simulink model "v00_0A_0E"  (R2022b)
settings: Solver=FixedStepDiscrete  StartTime=0.0  StopTime=8000  FixedStep=SampleTime  MaxStep=Contactors_StepTime_msec  RelTol=1e-3  EnableMultiTasking=on
undefined symbols (not defined in the file): A_to_mA, BalancingTempGroup, canChannel, CapacityFactor, CC_Inputs, CellSOC, ChargeState, ContactorsFlags, DiscIntNeverNeededParam, gEN_Contactors_StepTime_msec, Ion, isDynamicCurrentEn, Lithium, maxAllowedImbalance, nCells_parallel, nCells_series, nCellTempGrps, PermanentFailRecoveryTrigger, ProtectionFlags, RBal_ohm, SampleTime, sigbuilder_block, StLineEq_varA, StLineEq_varB, TempSelectForDCL, Thresholds, V_to_mV
libraries: simulink x32, spsIdealSwitchLib x21, spsBatteryLib x20, spsSeriesRLCBranchLib x20, spsVoltageMeasurementLib x20, canmsglib x4, canlib x3, dspstat3 x2, spspowerguiLib x2, spsControlledCurrentSourceLib x1, spsCurrentMeasurementLib x1
(part 6 of 7)

== stateflow chart v00_0A_0E/Protection/CurrentVoltageTemperature_Statemachine ==
  state ThermalRunaway [parallel]
    settings: executionOrder=6
    state ThermalRunaway_Warning
      entry:
      ThermalRunaway = ProtectionFlags.Warning;
    state ThermalRunaway_NoError
      entry:
      ThermalRunaway = ProtectionFlags.NoError;
    state ThermalRunaway_PermanentFail
      entry:
      ThermalRunaway = ProtectionFlags.PermanentFail;
    state ThermalRunaway_Error
      entry:
      ThermalRunaway = ProtectionFlags.Error;
    ThermalRunaway_NoError -> ThermalRunaway_Warning : [duration((TempChange_C>=Thresholds.Protections_MaxAllowedTempChange_C && DataPipeline.TemperatureSenseBus(1).T_max >Thresholds.Protections_MaxOperatingTemp_C),msec) >=Thresholds.ThermalRunawayWarningTimeout_msec]
    (default) -> ThermalRunaway_NoError
    ThermalRunaway_Warning -> ThermalRunaway_Error : [duration((TempChange_C >= Thresholds.Protections_MaxAllowedTempChange_C && DataPipeline.TemperatureSenseBus(1).T_max > Thresholds.Protections_MaxOperatingTemp_C),msec) >=Thresholds.ThermalRunawayErrorTimeout_msec]
    ThermalRunaway_Error -> ThermalRunaway_PermanentFail : [duration((ThermalRunaway == ProtectionFlags.Error),msec) >=Thresholds.ThermalRunawayErrorTimeout_msec]
  state SuddenVoltageDrop [parallel]
    settings: executionOrder=10
    state Lobby
      entry:
      SuddenVoltageDrop = ProtectionFlags.NoError;
    state Error
      entry:
      SuddenVoltageDrop = ProtectionFlags.Error;
    (default) -> SuddenVoltageDrop.Lobby
    SuddenVoltageDrop.Lobby -> SuddenVoltageDrop.Error : [duration((VoltageDrop_mV >= Thresholds.Protections_SuddenVoltageDrop_mV_by_time),msec) >= Thresholds.SuddenVoltageDropTimeout_msec]
    SuddenVoltageDrop.Error -> SuddenVoltageDrop.Lobby : [duration((VoltageDrop_mV < Thresholds.Protections_SuddenVoltageDrop_mV_by_time),msec) >= Thresholds.SuddenVoltageDropTimeout_msec]
  state Current_Protection [parallel]
    settings: executionOrder=3
    state OCD_Error
      entry:
      OCDFlag = ProtectionFlags.Error;
      OCCFlag = ProtectionFlags.NoError;
    state Lobby
      entry:
      OCD_Warning_mA = Thresholds.Protections_OCD_Warning_mA;
      OCD_Error_mA = Thresholds.Protections_OCD_Error_mA;
      OCC_Warning_mA = Thresholds.Protections_OCC_Warning_mA;
      OCC_Error_mA = Thresholds.Protections_OCC_Error_mA;
    state OverCurrent_DynamicCurrentLimits
      entry:
      eFuseChargeFlag= ProtectionFlags.NoError;
      eFuseDischargeFlag= ProtectionFlags.NoError;
      during:
      i2tCalculation_DCL;
      DCL_Current_A = (single(DataPipeline.isChargeEn) * single(DataPipeline.DCL_ChargingCurrent_A))+(single(~DataPipeline.isChargeEn) * single(DataPipeline.DCL_DisChargingCurrent_A));
      state i2tCalculation_DCL [function]
        (default) -> (junction 1122) : % IfStatement
        (junction 1122) -> (junction 1125) [order 1] : [i2t_Calculated_A2sec >0]
        (junction 1125) -> (junction 1123) : {CurrentDiff_A = single(abs(DataPipeline.Current_mA)/1000) - single(abs(DCL_Current_A));
            | i2t_Calculated_A2sec = i2t_Calculated_A2sec - (CurrentDiff_A * CurrentDiff_A * DataPipeline.LoopTimer_SOC_msec/1000);}
        (junction 1122) -> (junction 1124) [order 2] : {i2t_Calculated_A2sec = single(0);}
        (junction 1123) -> (junction 1124)
        (junction 1124) -> (junction 1126)
    state OCD_Warning
      entry:
      OCDFlag = ProtectionFlags.Warning;
      OCCFlag = ProtectionFlags.NoError;
    state OCD_Recovery
      entry:
      OCDFlag = ProtectionFlags.Recovery;
      OCCFlag = ProtectionFlags.NoError;
    state No_Error_Current
      entry:
      OCDFlag = ProtectionFlags.NoError;
      OCCFlag = ProtectionFlags.NoError;
    state eFuse_Melting
      du:  eFuseWarning;
      DCL_Current_A = single((single(DataPipeline.isChargeEn) * single(DataPipeline.DCL_ChargingCurrent_A))+(single(~DataPipeline.isChargeEn) * single(DataPipeline.DCL_DisChargingCurrent_A)));
      CurrentDiff_A = single(abs(DataPipeline.Current_mA)/1000) - single(abs(DCL_Current_A));
      i2t_Calculated_A2sec = i2t_Calculated_A2sec + (CurrentDiff_A * CurrentDiff_A * DataPipeline.LoopTimer_SOC_msec/1000);
      % i2t_Calculated_A2sec = 110000;
      state eFuseWarning [function]
        (default) -> (junction 1136) : % eFuseDuringCharge&Discharge
        (junction 1136) -> (junction 1135) [order 1] : [DataPipeline.VCU.isChargerConnected == 1]
        (junction 1136) -> (junction 1139) [order 2] : {eFuseDischargeFlag= ProtectionFlags.Warning;}
        (junction 1135) -> (junction 1132) : {eFuseChargeFlag= ProtectionFlags.Warning;}
        (junction 1132) -> (junction 1139)
        (junction 1139) -> (junction 1138)
    state OCC_Warning
      entry:
      OCCFlag = ProtectionFlags.Warning;
      OCDFlag = ProtectionFlags.NoError;
    state OCC_Recovery
      entry:
      OCCFlag = ProtectionFlags.Recovery;
      OCDFlag = ProtectionFlags.NoError;
    state OCC_Error
      entry:
      OCCFlag = ProtectionFlags.Error;
      OCDFlag = ProtectionFlags.NoError;
    state eFuse_Melted
      entry:
      i2t_Calculated_A2sec = single(0);
      eFuseError;
      state eFuseError [function]
        (default) -> (junction 1146) : % eFuseDuringCharge&Discharge
        (junction 1146) -> (junction 1147) [order 1] : [DataPipeline.VCU.isChargerConnected == 1]
        (junction 1146) -> (junction 1148) [order 2] : {eFuseDischargeFlag= ProtectionFlags.Error;}
        (junction 1147) -> (junction 1149) : {eFuseChargeFlag= ProtectionFlags.Error;}
        (junction 1149) -> (junction 1148)
        (junction 1148) -> (junction 1153)
    state PermanentFail_eFuse
      entry:
      eFusePermanentFail;
      state eFusePermanentFail [function]
        (default) -> (junction 1167) : % eFuseDuringCharge&Discharge
        (junction 1167) -> (junction 1161) [order 1] : [DataPipeline.VCU.isChargerConnected == 1]
        (junction 1167) -> (junction 1170) [order 2] : {eFuseDischargeFlag= ProtectionFlags.PermanentFail;}
        (junction 1161) -> (junction 1164) : {eFuseChargeFlag= ProtectionFlags.PermanentFail;}
        (junction 1164) -> (junction 1170)
        (junction 1170) -> (junction 1165)
    (default) -> Current_Protection.Lobby
    OCD_Recovery -> OCD_Error [order 2] : [(duration(abs(DataPipeline.Current_mA) >= OCD_Error_mA, msec) > Thresholds.Protections_OCD_WarningTimeout_msec)]
    OCD_Warning -> OCD_Error [order 1] : [(duration(abs(DataPipeline.Current_mA) >= OCD_Error_mA, msec) > Thresholds.Protections_OCD_WarningTimeout_msec)]
    OCD_Error -> OCD_Recovery : [after(Thresholds.Protections_OCD_ErrorTimeout_msec, msec)]
    Current_Protection.Lobby -> No_Error_Current [order 2] : [DataPipeline.isDynamicCurrentEn == 0 ]
    Current_Protection.Lobby -> OverCurrent_DynamicCurrentLimits [order 1] : [DataPipeline.isDynamicCurrentEn == 1 ]
    No_Error_Current -> OCD_Warning [order 1] : [DataPipeline.VCU.isChargerConnected == 0 && duration(abs(DataPipeline.Current_mA) >= OCD_Warning_mA, msec) > Thresholds.Protections_OCD_NoErrorTimeout_msec]
    OCD_Warning -> No_Error_Current [order 2] : [duration(abs(DataPipeline.Current_mA) <= OCD_Warning_mA, msec) > Thresholds.Protections_OCD_WarningTimeout_msec]
    OCD_Recovery -> No_Error_Current [order 1] : [duration(abs(DataPipeline.Current_mA) <= OCD_Error_mA, msec) > Thresholds.Protections_OCD_RecoveryTimeout_msec]
    eFuse_Melted -> OverCurrent_DynamicCurrentLimits [order 1] : [after(Thresholds.i2tTimeout_msec,msec)]
    OCC_Recovery -> No_Error_Current [order 1] : [duration(abs(DataPipeline.Current_mA) <= OCC_Error_mA, msec) > Thresholds.Protections_OCC_RecoveryTimeout_msec]
    No_Error_Current -> OCC_Warning [order 2] : [DataPipeline.VCU.isChargerConnected == 1 && duration(abs(DataPipeline.Current_mA) >= OCC_Warning_mA,msec) > Thresholds.Protections_OCC_NoErrorTimeout_msec]
    OCC_Warning -> No_Error_Current [order 2] : [duration(abs(DataPipeline.Current_mA) <= OCC_Warning_mA, msec) > Thresholds.Protections_OCC_WarningTimeout_msec]
    OverCurrent_DynamicCurrentLimits -> eFuse_Melting : [duration((abs(DataPipeline.Current_mA)/1000) > abs(DCL_Current_A),msec) >= Thresholds.i2tTimeout_msec]
    eFuse_Melting -> OverCurrent_DynamicCurrentLimits [order 1] : [duration((abs(DataPipeline.Current_mA)/1000) < abs(DCL_Current_A),msec) >= Thresholds.i2tTimeout_msec]
    OCC_Warning -> OCC_Error [order 1] : [duration(abs(DataPipeline.Current_mA) >= OCC_Error_mA, msec) > Thresholds.Protections_OCC_WarningTimeout_msec]
    OCC_Error -> OCC_Recovery : [after(Thresholds.Protections_OCC_ErrorTimeout_msec, msec)]
    OCC_Recovery -> OCC_Error [order 2] : [duration(abs(DataPipeline.Current_mA) >= OCC_Error_mA, msec) > Thresholds.Protections_OCC_WarningTimeout_msec]
    eFuse_Melting -> eFuse_Melted [order 2] : [duration(((i2t_Calculated_A2sec >= DataPipeline.i2t_ChargingCurrent_A2sec && DataPipeline.VCU.isChargerConnected == 1)), msec)>= Thresholds.eFuseMeltingTimeout_msec || duration(((i2t_Calculated_A2sec >= DataPipeline.i2t_DisChargingCurrent_A2sec && DataPipeline.VCU.isChargerConnected == 0)), msec)>= Thresholds.eFuseMeltingTimeout_msec]
        | {eFuseMeltCount = eFuseMeltCount + 1;}
    eFuse_Melted -> PermanentFail_eFuse [order 2] : [eFuseMeltCount >= Thresholds.PermanentFailCounts_eFuse]
  state Voltage_Protection [parallel]
    settings: executionOrder=2
    state UV_Error
      entry:
      UVFlag = ProtectionFlags.Error;
      OVFlag = ProtectionFlags.NoError;
    state UV_Recovery
      entry:
      UVFlag = ProtectionFlags.Recovery;
      OVFlag = ProtectionFlags.NoError;
    state UV_Warning
      entry:
      UVFlag = ProtectionFlags.Warning;
      OVFlag = ProtectionFlags.NoError;
    state No_Error_Voltage
      entry:
      UVFlag = ProtectionFlags.NoError;
      OVFlag = ProtectionFlags.NoError;
    state OV_Recovery
      entry:
      OVFlag = ProtectionFlags.Recovery;
      UVFlag = ProtectionFlags.NoError;
    state OV_Warning
      entry:
      OVFlag = ProtectionFlags.Warning;
      UVFlag = ProtectionFlags.NoError;
    state OV_Error
      entry:
      OVFlag = ProtectionFlags.Error;
      UVFlag = ProtectionFlags.NoError;
    UV_Recovery -> UV_Error [order 2] : [duration((DataPipeline.VoltageSenseBus.mV_min < Thresholds.Protections_UV_Error_mV), msec) > Thresholds.Protections_UV_WarningTimeout_msec]
    UV_Warning -> UV_Error [order 2] : [duration((DataPipeline.VoltageSenseBus.mV_min < Thresholds.Protections_UV_Error_mV && DataPipeline.VCU.isChargerConnected == 0), msec) > Thresholds.Protections_UV_WarningTimeout_msec]
    UV_Error -> UV_Recovery : [(duration((DataPipeline.VoltageSenseBus.mV_min > Thresholds.Protections_UV_Error_mV  || DataPipeline.VCU.isChargerConnected ==1), msec) > Thresholds.Protections_UV_ErrorTimeout_msec)]
    No_Error_Voltage -> UV_Warning [order 1] : [(duration(DataPipeline.VoltageSenseBus.mV_min <= Thresholds.Protections_UV_Warning_mV, msec) > Thresholds.Protections_UV_NoErrorTimeout_msec)]
    UV_Warning -> No_Error_Voltage [order 1] : [(duration((DataPipeline.VoltageSenseBus.mV_min > Thresholds.Protections_UV_Warning_mV), msec) > Thresholds.Protections_OV_WarningTimeout_msec)]
    UV_Recovery -> No_Error_Voltage [order 1] : [duration((DataPipeline.VoltageSenseBus.mV_min >= Thresholds.Protections_UV_Recovery_mV || DataPipeline.VCU.isChargerConnected ==1),msec) > Thresholds.Protections_UV_RecoveryTimeout_msec]
    (default) -> No_Error_Voltage
    No_Error_Voltage -> OV_Warning [order 2] : [duration(DataPipeline.VoltageSenseBus.mV_max >= Protections_OV_Warning_mV && (DataPipeline.VCU.isChargerConnected==1 || DataPipeline.Current_mA>0), msec) > Thresholds.Protections_OV_NoErrorTimeout_msec]
    OV_Recovery -> No_Error_Voltage [order 1] : [duration((DataPipeline.VoltageSenseBus.mV_max <= Protections_OV_Recovery_mV || DataPipeline.VCU.isChargerConnected ==0), msec) > Thresholds.Protections_OV_RecoveryTimeout_msec]
    OV_Warning -> No_Error_Voltage [order 1] : [(duration((DataPipeline.VoltageSenseBus.mV_max < Protections_OV_Warning_mV), msec) > Thresholds.Protections_OV_WarningTimeout_msec)]
    OV_Error -> OV_Recovery : [(duration((DataPipeline.VoltageSenseBus.mV_max < Protections_OV_Error_mV || DataPipeline.VCU.isChargerConnected ==0), msec) > Thresholds.Protections_OV_ErrorTimeout_msec)]
    OV_Recovery -> OV_Error [order 2] : [(duration((DataPipeline.VoltageSenseBus.mV_max > Protections_OV_Error_mV), msec) > Thresholds.Protections_OV_WarningTimeout_msec)]
    OV_Warning -> OV_Error [order 2] : [duration(DataPipeline.VoltageSenseBus.mV_max > Protections_OV_Error_mV && (DataPipeline.VCU.isChargerConnected ==1 || DataPipeline.Current_mA>0), msec) > Thresholds.Protections_OV_WarningTimeout_msec]
  state TemperatureGradient [parallel]
    settings: executionOrder=7
    state Lobby
      entry:
      TemperatureGradient = ProtectionFlags.NoError;
    state Error
      entry:
      TemperatureGradient = ProtectionFlags.Error;
    (default) -> TemperatureGradient.Lobby
    TemperatureGradient.Error -> TemperatureGradient.Lobby : [duration(DataPipeline.DeltaTemperatureGroup1_C < Thresholds.Protections_MaxAllowedTempGradientGroup1_C, msec) >= Thresholds.TemperatureGradientTimeout_msec]
    TemperatureGradient.Lobby -> TemperatureGradient.Error : [duration(DataPipeline.DeltaTemperatureGroup1_C >= Thresholds.Protections_MaxAllowedTempGradientGroup1_C, msec) >= Thresholds.TemperatureGradientTimeout_msec]
  state OverallState [parallel]
    settings: executionOrder=12
    state Lobby
      entry: TempOverallState = ProtectionFlags.NoError;
    state Warning
      entry: TempOverallState = ProtectionFlags.Warning;
    state Error
      entry: TempOverallState = ProtectionFlags.Error;
    state Recovery
      entry:  TempOverallState = ProtectionFlags.Recovery;
    (default) -> OverallState.Lobby
    Warning -> OverallState.Lobby [order 2] : [FlagGroup1 == 0 && FlagGroup2 == 0]
    OverallState.Lobby -> Warning : [FlagGroup1 >= 1 || FlagGroup2 >= 1]
    OverallState.Error -> OverallState.Lobby [order 2] : [FlagGroup1 == 0 && FlagGroup2 == 0]
    Recovery -> OverallState.Lobby : [FlagGroup1 == 0 && FlagGroup2 == 0]
    Warning -> OverallState.Error [order 1] : [FlagGroup1 >= 2 || FlagGroup2 >= 2]
    OverallState.Error -> Recovery [order 1] : [(FlagGroup1 == 3 && FlagGroup2 == 0)||(FlagGroup1 == 0 && FlagGroup2==3)]
  state HighImbalanceFlag [parallel]
    settings: executionOrder=8
    state Lobby
      entry:
      HighImbalanceFlag = ProtectionFlags.NoError;
    state Error
      entry:
      HighImbalanceFlag = ProtectionFlags.Error;
    (default) -> HighImbalanceFlag.Lobby
    HighImbalanceFlag.Lobby -> HighImbalanceFlag.Error : [duration((DataPipeline.VoltageSenseBus.VoltageDelta_mV >= Thresholds.Protections_HighImbalanceError_mV),msec) >= Thresholds.HighImbalanceFlagTimeout_msec]
    HighImbalanceFlag.Error -> HighImbalanceFlag.Lobby : [duration((DataPipeline.VoltageSenseBus.VoltageDelta_mV < Thresholds.Protections_HighImbalanceError_mV),msec) >= Thresholds.HighImbalanceFlagTimeout_msec]
  state ErrorDetect [parallel]
    settings: executionOrder=11
    state Lobby
      entry:
      ErrorDetect = ProtectionFlags.NoError;
    state Error
      entry:
      ErrorDetect = ProtectionFlags.Error;
    (default) -> ErrorDetect.Lobby
    ErrorDetect.Lobby -> ErrorDetect.Error : [ThermalRunaway==ProtectionFlags.Error||TemperatureGradient==ProtectionFlags.Error||HighImbalanceFlag==ProtectionFlags.Error||ShortCircuitDetect==ProtectionFlags.Error||SuddenVoltageDrop == ProtectionFlags.Error||TempOverallState==ProtectionFlags.Error||OCCFlag==ProtectionFlags.Error||OCDFlag==ProtectionFlags.Error||UVFlag==ProtectionFlags.Error||OVFlag==ProtectionFlags.Error ||eFuseChargeFlag==ProtectionFlags.Error || eFuseDischargeFlag==ProtectionFlags.Error]
    ErrorDetect.Error -> ErrorDetect.Lobby : [ThermalRunaway~=ProtectionFlags.Error && TemperatureGradient~=ProtectionFlags.Error && HighImbalanceFlag~=ProtectionFlags.Error && ShortCircuitDetect~=ProtectionFlags.Error && SuddenVoltageDrop~=ProtectionFlags.Error && TempOverallState~=ProtectionFlags.Error && OCCFlag~=ProtectionFlags.Error && OCDFlag~=ProtectionFlags.Error && UVFlag~=ProtectionFlags.Error && OVFlag~=ProtectionFlags.Error && eFuseChargeFlag~=ProtectionFlags.Error && eFuseDischargeFlag~=ProtectionFlags.Error]
  state ShortCircuitDetect [parallel]
    settings: executionOrder=9
    state Lobby
      entry:
      ShortCircuitDetect = ProtectionFlags.NoError;
    state Error
      entry:
      ShortCircuitDetect = ProtectionFlags.Error;
    (default) -> ShortCircuitDetect.Lobby
    ShortCircuitDetect.Lobby -> ShortCircuitDetect.Error : [duration((abs(DataPipeline.Current_mA) >= Thresholds.Protections_ShortCircuitCurrent_mA),msec) >= Thresholds.ShortCircuitDetect_msec]
    ShortCircuitDetect.Error -> ShortCircuitDetect.Lobby : [duration((abs(DataPipeline.Current_mA) < Thresholds.Protections_ShortCircuitCurrent_mA),msec) >= Thresholds.ShortCircuitDetect_msec]
  state OVThresholds_Selection [parallel]
    settings: executionOrder=1
    state SlowCharge_OVThrs_Selection
      entry: Protections_OV_Warning_mV = Thresholds.Protections_SlowCh_OV_Warning_mV;
      Protections_OV_Error_mV = Thresholds.Protections_SlowCh_OV_Error_mV;
      Protections_OV_Recovery_mV = Thresholds.Protections_SlowCh_OV_Recovery_mV;
    state FastCharge_OVThrs_Selection
      entry: Protections_OV_Warning_mV = Thresholds.Protections_FastCh_OV_Warning_mV;
      Protections_OV_Error_mV = Thresholds.Protections_FastCh_OV_Error_mV;
      Protections_OV_Recovery_mV = Thresholds.Protections_FastCh_OV_Recovery_mV;
    (default) -> SlowCharge_OVThrs_Selection
    SlowCharge_OVThrs_Selection -> FastCharge_OVThrs_Selection : [DataPipeline.VCU.isChargerConnected == true && DataPipeline.VCU.FastCharge == true]
    FastCharge_OVThrs_Selection -> SlowCharge_OVThrs_Selection : [DataPipeline.VCU.isChargerConnected == false || DataPipeline.VCU.FastCharge == false]
  state DCL_CurrentProtection [parallel]
    settings: executionOrder=13
    state DCL_Protection_Lobby
      en:
      TimeReset = 0;
      DCLI_CurrentFlag = ProtectionFlags.NoError;
      DCLO_CurrentFlag = ProtectionFlags.NoError;
    state IntState
      en:
    state DCLI_Warning
      en:
      TimeReset = 1;
      DCLI_CurrentFlag = ProtectionFlags.Warning;
    state DCLI_Error
      entry:
      DCLI_CurrentFlag = ProtectionFlags.Error;
    state IntStat1
      en:
    state IntStat2
      en:
    state IntStat3
      en:
    state IntStat4
      en:
    state IntStat5
      en:
    state DCLO_Warning
      entry:
      TimeReset = 1;
      DCLO_CurrentFlag = ProtectionFlags.Warning;
    state DCLO_Error
      entry:
      DCLO_CurrentFlag = ProtectionFlags.Error;
    (default) -> DCL_Protection_Lobby
    DCL_Protection_Lobby -> IntState [order 2] : [DataPipeline.VCU.isChargerConnected == 1 && abs(DataPipeline.Current_mA/1000)>DataPipeline.DCL_ChargingCurrent_A]{TimeReset = 1;}
    IntState -> DCLI_Warning [order 1] : [IntegratedTime>Thresholds.DCL_CurrentProtectionTimeout_msec]{TimeReset = 0;}
    DCLI_Warning -> DCLI_Error [order 2] : [IntegratedTime>Thresholds.DCL_WarningToErrorTimeout_msec]{TimeReset=0;}
    IntState -> DCL_Protection_Lobby [order 2] : [DataPipeline.VCU.isChargerConnected ~= 1 || abs(DataPipeline.Current_mA/1000)<DataPipeline.DCL_ChargingCurrent_A]
    DCLI_Warning -> IntStat1 [order 1] : [DataPipeline.VCU.isChargerConnected ~= 1 || abs(DataPipeline.Current_mA/1000)<DataPipeline.DCL_ChargingCurrent_A]{TimeReset = 1;}
    IntStat1 -> DCL_Protection_Lobby [order 1] : [IntegratedTime>Thresholds.DCL_CurrentProtectionTimeout_msec]{TimeReset = 0;}
    IntStat1 -> DCLI_Warning [order 2] : [DataPipeline.VCU.isChargerConnected == 1 || abs(DataPipeline.Current_mA/1000)>DataPipeline.DCL_ChargingCurrent_A]{TimeReset = 0;}
    IntStat2 -> DCLI_Error [order 2] : [DataPipeline.VCU.isChargerConnected == 1 && abs(DataPipeline.Current_mA/1000)>DataPipeline.DCL_ChargingCurrent_A]
    IntStat2 -> DCL_Protection_Lobby [order 1] : [IntegratedTime>Thresholds.DCL_RecoveryCurrentProtectionTimeout_msec]{TimeReset = 0;}
    DCLI_Error -> IntStat2 : [DataPipeline.VCU.isChargerConnected ~= 1 || abs(DataPipeline.Current_mA/1000)<DataPipeline.DCL_ChargingCurrent_A]{TimeReset = 1;}
    DCL_Protection_Lobby -> IntStat3 [order 1] : [DataPipeline.VCU.isChargerConnected == 0 && abs(DataPipeline.Current_mA/1000)>DataPipeline.DCL_DisChargingCurrent_A]{TimeReset = 1;}
    IntStat3 -> DCL_Protection_Lobby [order 2] : [DataPipeline.VCU.isChargerConnected ~= 0 || abs(DataPipeline.Current_mA/1000)<DataPipeline.DCL_DisChargingCurrent_A]{TimeReset = 0;}
    IntStat5 -> DCL_Protection_Lobby [order 1] : [IntegratedTime>Thresholds.DCL_RecoveryCurrentProtectionTimeout_msec]{TimeReset = 0;}
    IntStat4 -> DCL_Protection_Lobby [order 1] : [IntegratedTime>Thresholds.DCL_CurrentProtectionTimeout_msec]{TimeReset = 0;}
    DCLO_Error -> IntStat5 : [DataPipeline.VCU.isChargerConnected ~= 0 || abs(DataPipeline.Current_mA/1000)<DataPipeline.DCL_DisChargingCurrent_A]{TimeReset = 1;}
    IntStat3 -> DCLO_Warning [order 1] : [IntegratedTime>Thresholds.DCL_CurrentProtectionTimeout_msec]{TimeReset = 0;}
    DCLO_Warning -> IntStat4 [order 1] : [DataPipeline.VCU.isChargerConnected ~= 0 || abs(DataPipeline.Current_mA/1000)<DataPipeline.DCL_DisChargingCurrent_A]{TimeReset = 1;}
    IntStat4 -> DCLO_Warning [order 2] : [DataPipeline.VCU.isChargerConnected == 0 && abs(DataPipeline.Current_mA/1000)<DataPipeline.DCL_DisChargingCurrent_A]{TimeReset = 0;}
    IntStat5 -> DCLO_Error [order 2] : [DataPipeline.VCU.isChargerConnected == 0 && abs(DataPipeline.Current_mA/1000)>DataPipeline.DCL_DisChargingCurrent_A]{TimeReset = 0;}
    DCLO_Warning -> DCLO_Error [order 2] : [IntegratedTime>Thresholds.DCL_WarningToErrorTimeout_msec]{TimeReset=0;}
  state Temperature_Protection_Group1 [parallel]
    settings: executionOrder=4
    state UTD_Error
      entry:
      FlagGroup1 = ProtectionFlags.Error;
      TempState1 = TempState.UTD;
    state UTC_Error
      entry:
      FlagGroup1 = ProtectionFlags.Error;
      TempState1 = TempState.UTC;
    state UTD_Recovery
      entry:
      FlagGroup1 = ProtectionFlags.Recovery;
      TempState1 = TempState.UTD;
    state UTD_Warning
      entry:
      FlagGroup1 = ProtectionFlags.Warning;
      TempState1 = TempState.UTD;
    state UTC_Recovery
      entry:
      FlagGroup1 = ProtectionFlags.Recovery;
      TempState1 = TempState.UTC;
    state UTC_Warning
      entry:
      FlagGroup1 = ProtectionFlags.Warning;
      TempState1 = TempState.UTC;
    state No_Error_Temperature
      entry:
      FlagGroup1 = ProtectionFlags.NoError;
      TempState1 = TempState.NoErr;
    state OTC_Recovery
      entry:
      FlagGroup1 = ProtectionFlags.Recovery;
      TempState1 = TempState.OTC;
    state OTC_Warning
      entry:
      FlagGroup1 = ProtectionFlags.Warning;
      TempState1 = TempState.OTC;
    state OTD_Recovery
      entry:
      FlagGroup1 = ProtectionFlags.Recovery;
      TempState1 = TempState.OTD;
    state OTD_Warning
      entry:
      FlagGroup1 = ProtectionFlags.Warning;
      TempState1 = TempState.OTD;
    state OTC_Error
      entry:
      FlagGroup1 = ProtectionFlags.Error;
      TempState1 = TempState.OTC;
    state OTD_Error
      entry:
      FlagGroup1 = ProtectionFlags.Error;
      TempState1 = TempState.OTD;
    Temperature_Protection_Group1.UTD_Recovery -> Temperature_Protection_Group1.UTD_Error [order 2] : [duration(DataPipeline.TemperatureSenseBus(1).T_min <= Thresholds.Temperature(1).Protections_UTD_Error_C,msec)>Thresholds.Temperature(1).Protections_UTD_WarningTimeout_msec]
    Temperature_Protection_Group1.UTD_Warning -> Temperature_Protection_Group1.UTD_Error [order 1] : [duration(DataPipeline.TemperatureSenseBus(1).T_min <= Thresholds.Temperature(1).Protections_UTD_Error_C,msec)>Thresholds.Temperature(1).Protections_UTD_WarningTimeout_msec]
    Temperature_Protection_Group1.UTD_Error -> Temperature_Protection_Group1.UTD_Recovery : [duration(DataPipeline.TemperatureSenseBus(1).T_min >= Thresholds.Temperature(1).Protections_UTD_Error_C,msec)>=Thresholds.Temperature(1).Protections_UTD_ErrorTimeout_msec]
    Temperature_Protection_Group1.UTC_Warning -> Temperature_Protection_Group1.UTC_Error [order 1] : [duration(DataPipeline.TemperatureSenseBus(1).T_min <= Thresholds.Temperature(1).Protections_UTC_Error_C,msec)>=Thresholds.Temperature(1).Protections_UTC_WarningTimeout_msec]
    Temperature_Protection_Group1.UTC_Recovery -> Temperature_Protection_Group1.UTC_Error [order 2] : [duration(DataPipeline.TemperatureSenseBus(1).T_min <= Thresholds.Temperature(1).Protections_UTC_Error_C,msec)>=Thresholds.Temperature(1).Protections_UTC_WarningTimeout_msec]
    Temperature_Protection_Group1.UTC_Error -> Temperature_Protection_Group1.UTC_Recovery : [duration(DataPipeline.TemperatureSenseBus(1).T_min >= Thresholds.Temperature(1).Protections_UTC_Error_C,msec)>=Thresholds.Temperature(1).Protections_UTC_ErrorTimeout_msec]
    Temperature_Protection_Group1.UTD_Recovery -> Temperature_Protection_Group1.No_Error_Temperature [order 1] : [duration(DataPipeline.TemperatureSenseBus(1).T_min >= Thresholds.Temperature(1).Protections_UTD_Recovery_C,msec)>=Thresholds.Temperature(1).Protections_UTD_RecoveryTimeout_msec]
    Temperature_Protection_Group1.UTD_Warning -> Temperature_Protection_Group1.No_Error_Temperature [order 2] : [duration(DataPipeline.TemperatureSenseBus(1).T_min >= Thresholds.Temperature(1).Protections_UTD_Warning_C,msec)>=Thresholds.Temperature(1).Protections_UTD_WarningTimeout_msec]
    Temperature_Protection_Group1.No_Error_Temperature -> Temperature_Protection_Group1.UTD_Warning [order 4] : [duration(DataPipeline.TemperatureSenseBus(1).T_min <= Thresholds.Temperature(1).Protections_UTD_Warning_C,msec)>=Thresholds.Temperature(1).Protections_UTD_NoErrorTimeout_msec && DataPipeline.VCU.isChargerConnected == 0]
    Temperature_Protection_Group1.No_Error_Temperature -> Temperature_Protection_Group1.UTC_Warning [order 1] : [duration(DataPipeline.TemperatureSenseBus(1).T_min <= Thresholds.Temperature(1).Protections_UTC_Warning_C,msec)>= Thresholds.Temperature(1).Protections_UTC_NoErrorTimeout_msec && DataPipeline.VCU.isChargerConnected == 1]
    Temperature_Protection_Group1.UTC_Warning -> Temperature_Protection_Group1.No_Error_Temperature [order 2] : [duration(DataPipeline.TemperatureSenseBus(1).T_min >= Thresholds.Temperature(1).Protections_UTC_Warning_C,msec)>=Thresholds.Temperature(1).Protections_UTC_WarningTimeout_msec]
    Temperature_Protection_Group1.UTC_Recovery -> Temperature_Protection_Group1.No_Error_Temperature [order 1] : [duration(DataPipeline.TemperatureSenseBus(1).T_min >= Thresholds.Temperature(1).Protections_UTC_Recovery_C,msec)>=Thresholds.Temperature(1).Protections_UTC_RecoveryTimeout_msec]
    (default) -> Temperature_Protection_Group1.No_Error_Temperature
    Temperature_Protection_Group1.No_Error_Temperature -> Temperature_Protection_Group1.OTD_Warning [order 3] : [duration(DataPipeline.TemperatureSenseBus(1).T_max >= Thresholds.Temperature(1).Protections_OTD_Warning_C,msec)>=Thresholds.Temperature(1).Protections_OTD_NoErrorTimeout_msec && DataPipeline.VCU.isChargerConnected == 0]
    Temperature_Protection_Group1.OTD_Warning -> Temperature_Protection_Group1.No_Error_Temperature [order 2] : [duration(DataPipeline.TemperatureSenseBus(1).T_max <= Thresholds.Temperature(1).Protections_OTD_Warning_C,msec)>=Thresholds.Temperature(1).Protections_OTD_WarningTimeout_msec]
    Temperature_Protection_Group1.OTD_Recovery -> Temperature_Protection_Group1.No_Error_Temperature [order 1] : [duration(DataPipeline.TemperatureSenseBus(1).T_max <= Thresholds.Temperature(1).Protections_OTD_Recovery_C,msec)>=Thresholds.Temperature(1).Protections_OTD_RecoveryTimeout_msec]
    Temperature_Protection_Group1.No_Error_Temperature -> Temperature_Protection_Group1.OTC_Warning [order 2] : [duration(DataPipeline.TemperatureSenseBus(1).T_max >= Thresholds.Temperature(1).Protections_OTC_Warning_C,msec)>=Thresholds.Temperature(1).Protections_OTC_NoErrorTimeout_msec && DataPipeline.VCU.isChargerConnected == 1]
    Temperature_Protection_Group1.OTC_Recovery -> Temperature_Protection_Group1.No_Error_Temperature [order 1] : [duration(DataPipeline.TemperatureSenseBus(1).T_max <= Thresholds.Temperature(1).Protections_OTC_Recovery_C,msec)>=Thresholds.Temperature(1).Protections_OTC_RecoveryTimeout_msec]
    Temperature_Protection_Group1.OTC_Warning -> Temperature_Protection_Group1.No_Error_Temperature [order 1] : [duration(DataPipeline.TemperatureSenseBus(1).T_max <= Thresholds.Temperature(1).Protections_OTC_Warning_C,msec)>=Thresholds.Temperature(1).Protections_OTC_WarningTimeout_msec]
    Temperature_Protection_Group1.OTC_Warning -> Temperature_Protection_Group1.OTC_Error [order 2] : [duration(DataPipeline.TemperatureSenseBus(1).T_max >= Thresholds.Temperature(1).Protections_OTC_Error_C,msec)>=Thresholds.Temperature(1).Protections_OTC_WarningTimeout_msec]
    Temperature_Protection_Group1.OTC_Error -> Temperature_Protection_Group1.OTC_Recovery : [duration(DataPipeline.TemperatureSenseBus(1).T_max <= Thresholds.Temperature(1).Protections_OTC_Error_C,msec)>=Thresholds.Temperature(1).Protections_OTC_ErrorTimeout_msec]
    Temperature_Protection_Group1.OTC_Recovery -> Temperature_Protection_Group1.OTC_Error [order 2] : [duration(DataPipeline.TemperatureSenseBus(1).T_max >= Thresholds.Temperature(1).Protections_OTC_Error_C,msec)>=Thresholds.Temperature(1).Protections_OTC_WarningTimeout_msec]
    Temperature_Protection_Group1.OTD_Error -> Temperature_Protection_Group1.OTD_Recovery : [duration(DataPipeline.TemperatureSenseBus(1).T_max <= Thresholds.Temperature(1).Protections_OTD_Error_C,msec)>=Thresholds.Temperature(1).Protections_OTD_ErrorTimeout_msec]
    Temperature_Protection_Group1.OTD_Recovery -> Temperature_Protection_Group1.OTD_Error [order 2] : [duration(DataPipeline.TemperatureSenseBus(1).T_max >= Thresholds.Temperature(1).Protections_OTD_Error_C,msec)>=Thresholds.Temperature(1).Protections_OTD_WarningTimeout_msec]
    Temperature_Protection_Group1.OTD_Warning -> Temperature_Protection_Group1.OTD_Error [order 1] : [duration(DataPipeline.TemperatureSenseBus(1).T_max >= Thresholds.Temperature(1).Protections_OTD_Error_C,msec)>=Thresholds.Temperature(1).Protections_OTD_WarningTimeout_msec]
  state Temperature_Protection_Group2 [parallel]
    settings: executionOrder=5
    state UTD_Error
      entry:
      FlagGroup2 = ProtectionFlags.Error;
      TempState2 = TempState.UTD;
    state UTC_Error
      entry:
      FlagGroup2 = ProtectionFlags.Error;
      TempState2 = TempState.UTC;
    state UTD_Warning
      entry:
      FlagGroup2 = ProtectionFlags.Warning;
      TempState2 = TempState.UTD;
    state UTD_Recovery
      entry:
      FlagGroup2 = ProtectionFlags.Recovery;
      TempState2 = TempState.UTD;
    state UTC_Warning
      entry:
      FlagGroup2 = ProtectionFlags.Warning;
      TempState2 = TempState.UTC;
    state UTC_Recovery
      entry:
      FlagGroup2 = ProtectionFlags.Recovery;
      TempState2 = TempState.UTC;
    state No_Error_Temperature
      entry:
      FlagGroup2 = ProtectionFlags.NoError;
      TempState2 = TempState.NoErr;
    state OTC_Recovery
      entry:
      FlagGroup2 = ProtectionFlags.Recovery;
      TempState2 = TempState.OTC;
    state OTC_Warning
      entry:
      FlagGroup2 = ProtectionFlags.Warning;
      TempState2 = TempState.OTC;
    state OTD_Recovery
      entry:
      FlagGroup2 = ProtectionFlags.Recovery;
      TempState2 = TempState.OTD;
    state OTD_Warning
      entry:
      FlagGroup2 = ProtectionFlags.Warning;
      TempState2 = TempState.OTD;
    state OTC_Error
      entry:
      FlagGroup2 = ProtectionFlags.Error;
      TempState2 = TempState.OTC;
    state OTD_Error
      entry:
      FlagGroup2 = ProtectionFlags.Error;
      TempState2 = TempState.OTD;
    Temperature_Protection_Group2.UTD_Recovery -> Temperature_Protection_Group2.UTD_Error [order 2] : [duration(DataPipeline.TemperatureSenseBus(2).T_min <= Thresholds.Temperature(2).Protections_UTD_Error_C,msec)>=Thresholds.Temperature(2).Protections_UTD_WarningTimeout_msec]
    Temperature_Protection_Group2.UTD_Warning -> Temperature_Protection_Group2.UTD_Error [order 1] : [duration(DataPipeline.TemperatureSenseBus(2).T_min <= Thresholds.Temperature(2).Protections_UTD_Error_C,msec)>=Thresholds.Temperature(2).Protections_UTD_WarningTimeout_msec]
    Temperature_Protection_Group2.UTD_Error -> Temperature_Protection_Group2.UTD_Recovery : [duration(DataPipeline.TemperatureSenseBus(2).T_min >= Thresholds.Temperature(2).Protections_UTD_Error_C,msec)>=Thresholds.Temperature(2).Protections_UTD_ErrorTimeout_msec]
    Temperature_Protection_Group2.UTC_Warning -> Temperature_Protection_Group2.UTC_Error [order 1] : [duration(DataPipeline.TemperatureSenseBus(2).T_min <= Thresholds.Temperature(2).Protections_UTC_Error_C,msec)>=Thresholds.Temperature(2).Protections_UTC_WarningTimeout_msec]
    Temperature_Protection_Group2.UTC_Recovery -> Temperature_Protection_Group2.UTC_Error [order 2] : [duration(DataPipeline.TemperatureSenseBus(2).T_min <= Thresholds.Temperature(2).Protections_UTC_Error_C,msec)>=Thresholds.Temperature(2).Protections_UTC_WarningTimeout_msec]
    Temperature_Protection_Group2.UTC_Error -> Temperature_Protection_Group2.UTC_Recovery : [duration(DataPipeline.TemperatureSenseBus(2).T_min >= Thresholds.Temperature(2).Protections_UTC_Error_C,msec)>=Thresholds.Temperature(2).Protections_UTC_ErrorTimeout_msec]
    Temperature_Protection_Group2.UTD_Warning -> Temperature_Protection_Group2.No_Error_Temperature [order 2] : [duration(DataPipeline.TemperatureSenseBus(2).T_min >= Thresholds.Temperature(2).Protections_UTD_Warning_C,msec)>=Thresholds.Temperature(2).Protections_UTD_WarningTimeout_msec]
    Temperature_Protection_Group2.No_Error_Temperature -> Temperature_Protection_Group2.UTD_Warning [order 4] : [duration(DataPipeline.TemperatureSenseBus(2).T_min <= Thresholds.Temperature(2).Protections_UTD_Warning_C,msec)>=Thresholds.Temperature(2).Protections_UTD_WarningTimeout_msec && DataPipeline.VCU.isChargerConnected == 0]
    Temperature_Protection_Group2.UTD_Recovery -> Temperature_Protection_Group2.No_Error_Temperature [order 1] : [duration(DataPipeline.TemperatureSenseBus(2).T_min >= Thresholds.Temperature(2).Protections_UTD_Recovery_C,msec)>=Thresholds.Temperature(2).Protections_UTD_RecoveryTimeout_msec]
    Temperature_Protection_Group2.No_Error_Temperature -> Temperature_Protection_Group2.UTC_Warning [order 1] : [duration(DataPipeline.TemperatureSenseBus(2).T_min <= Thresholds.Temperature(2).Protections_UTC_Warning_C,msec)>=Thresholds.Temperature(2).Protections_UTC_WarningTimeout_msec && DataPipeline.VCU.isChargerConnected == 1]
    Temperature_Protection_Group2.UTC_Warning -> Temperature_Protection_Group2.No_Error_Temperature [order 2] : [duration(DataPipeline.TemperatureSenseBus(2).T_min >= Thresholds.Temperature(2).Protections_UTC_Warning_C,msec)>=Thresholds.Temperature(2).Protections_UTC_WarningTimeout_msec]
    Temperature_Protection_Group2.UTC_Recovery -> Temperature_Protection_Group2.No_Error_Temperature [order 1] : [duration(DataPipeline.TemperatureSenseBus(2).T_min >= Thresholds.Temperature(2).Protections_UTC_Recovery_C,msec)>=Thresholds.Temperature(2).Protections_UTC_RecoveryTimeout_msec]
    (default) -> Temperature_Protection_Group2.No_Error_Temperature
    Temperature_Protection_Group2.No_Error_Temperature -> Temperature_Protection_Group2.OTD_Warning [order 3] : [duration(DataPipeline.TemperatureSenseBus(2).T_max >= Thresholds.Temperature(2).Protections_OTD_Warning_C,msec)>Thresholds.Temperature(2).Protections_OTD_WarningTimeout_msec && DataPipeline.VCU.isChargerConnected == 0]
    Temperature_Protection_Group2.OTD_Warning -> Temperature_Protection_Group2.No_Error_Temperature [order 2] : [duration(DataPipeline.TemperatureSenseBus(2).T_max <= Thresholds.Temperature(2).Protections_OTD_Warning_C,msec)>=Thresholds.Temperature(2).Protections_OTD_WarningTimeout_msec]
    Temperature_Protection_Group2.OTD_Recovery -> Temperature_Protection_Group2.No_Error_Temperature [order 1] : [duration(DataPipeline.TemperatureSenseBus(2).T_max <= Thresholds.Temperature(2).Protections_OTD_Recovery_C,msec)>=Thresholds.Temperature(2).Protections_OTD_RecoveryTimeout_msec]
    Temperature_Protection_Group2.No_Error_Temperature -> Temperature_Protection_Group2.OTC_Warning [order 2] : [duration(DataPipeline.TemperatureSenseBus(2).T_max >= Thresholds.Temperature(2).Protections_OTC_Warning_C,msec)>=Thresholds.Temperature(2).Protections_OTC_WarningTimeout_msec && DataPipeline.VCU.isChargerConnected == 1]
    Temperature_Protection_Group2.OTC_Recovery -> Temperature_Protection_Group2.No_Error_Temperature [order 1] : [duration(DataPipeline.TemperatureSenseBus(2).T_max <= Thresholds.Temperature(2).Protections_OTC_Recovery_C,msec)>=Thresholds.Temperature(2).Protections_OTC_RecoveryTimeout_msec]
    Temperature_Protection_Group2.OTC_Warning -> Temperature_Protection_Group2.No_Error_Temperature [order 1] : [duration(DataPipeline.TemperatureSenseBus(2).T_max <= Thresholds.Temperature(2).Protections_OTC_Warning_C,msec)>=Thresholds.Temperature(2).Protections_OTC_WarningTimeout_msec]
    Temperature_Protection_Group2.OTC_Warning -> Temperature_Protection_Group2.OTC_Error [order 2] : [duration(DataPipeline.TemperatureSenseBus(2).T_max >= Thresholds.Temperature(2).Protections_OTC_Error_C,msec)>=Thresholds.Temperature(2).Protections_OTC_WarningTimeout_msec]
    Temperature_Protection_Group2.OTC_Error -> Temperature_Protection_Group2.OTC_Recovery : [duration(DataPipeline.TemperatureSenseBus(2).T_max <= Thresholds.Temperature(2).Protections_OTC_Error_C,msec)>=Thresholds.Temperature(2).Protections_OTC_ErrorTimeout_msec]
    Temperature_Protection_Group2.OTC_Recovery -> Temperature_Protection_Group2.OTC_Error [order 2] : [duration(DataPipeline.TemperatureSenseBus(2).T_max >= Thresholds.Temperature(2).Protections_OTC_Error_C,msec)>=Thresholds.Temperature(2).Protections_OTC_WarningTimeout_msec]
    Temperature_Protection_Group2.OTD_Error -> Temperature_Protection_Group2.OTD_Recovery : [duration(DataPipeline.TemperatureSenseBus(2).T_max <= Thresholds.Temperature(2).Protections_OTD_Error_C,msec)>=Thresholds.Temperature(2).Protections_OTD_ErrorTimeout_msec]
    Temperature_Protection_Group2.OTD_Recovery -> Temperature_Protection_Group2.OTD_Error [order 2] : [duration(DataPipeline.TemperatureSenseBus(2).T_max >= Thresholds.Temperature(2).Protections_OTD_Error_C,msec)>=Thresholds.Temperature(2).Protections_OTD_WarningTimeout_msec]
    Temperature_Protection_Group2.OTD_Warning -> Temperature_Protection_Group2.OTD_Error [order 1] : [duration(DataPipeline.TemperatureSenseBus(2).T_max >= Thresholds.Temperature(2).Protections_OTD_Error_C,msec)>=Thresholds.Temperature(2).Protections_OTD_WarningTimeout_msec]
  data: TempChange_C input; VoltageDrop_mV input; Thresholds input; OCCFlag output Enum: ProtectionFlags =ProtectionFlags.NoError; OCDFlag output Enum: ProtectionFlags =ProtectionFlags.NoError; OVFlag output Enum: ProtectionFlags =ProtectionFlags.NoError; UVFlag output Enum: ProtectionFlags =ProtectionFlags.NoError; TempState2 output Enum: TempState; TempState1 output Enum: TempState; DataPipeline input; FlagGroup1 output; FlagGroup2 output; OCC_Error_mA local =int32(0); OCC_Warning_mA local =int32(0); OCD_Error_mA local =int32(0); OCD_Warning_mA local =int32(0); eFuseMeltCount local =uint8(0); ThermalRunaway output =ProtectionFlags.NoError; TemperatureGradient output; HighImbalanceFlag output; ShortCircuitDetect output; SuddenVoltageDrop output; ErrorDetect output; TempOverallState output; CurrentDiff_A local =single(0); DCL_Current_A local =single(0); i2t_Calculated_A2sec output =single(0); eFuseDischargeFlag output; eFuseChargeFlag output; Protections_OV_Recovery_mV local int32 =int32(3500); Protections_OV_Warning_mV local int32 =int32(3400); Protections_OV_Error_mV local int32 =int32(3600); DCLI_CurrentFlag output; DCLO_CurrentFlag output; IntegratedTime input; TimeReset output

== stateflow chart v00_0A_0E/CellBalancing/BalancingStateMachine ==
  state Terminate
    entry:
    BalanceFetCmd_AllOff;
    CurrentBalancingState = BalancingState.Terminate;
  state Lobby
    entry:
    CurrentBalancingState = BalancingState.Lobby;
  state Even_Balance
    entry:
    BalanceFetCmd_AllOff;
    CurrentBalancingState = BalancingState.Even_Balancing;
    exit:
    BalanceFetCmd_AllOff;
    state For_loop
      (default) -> (junction 24) : % For_loop
      (junction 24) -> (junction 26) : {i = 2;}
      (junction 26) -> (junction 25) [order 1] : [i<=nCells_series]
      (junction 28) -> (junction 26)
      (junction 26) -> (junction 29) [order 2]
      (junction 25) -> (junction 27) : {CellBalance(i);}
      (junction 27) -> (junction 28) : {i=i+2;}
  state BalanceFetCmd(index,cmd) [function]
    (default) -> (junction 64)
  state BalanceFetCmd_AllOff [function]
    (default) -> (junction 69) : {BalanceCmd(1:nCells_series) =0;}
  state Odd_Balance
    entry:
    BalanceFetCmd_AllOff;
    CurrentBalancingState = BalancingState.Odd_Balancing;
    exit:
    BalanceFetCmd_AllOff;
    state For_loop
      (default) -> (junction 129) : % For_loop
      (junction 129) -> (junction 130) : {i = 1;}
      (junction 130) -> (junction 131) [order 1] : [i<=nCells_series]
      (junction 134) -> (junction 130)
      (junction 130) -> (junction 132) [order 2]
      (junction 131) -> (junction 133) : {CellBalance(i);}
      (junction 133) -> (junction 134) : {i=i+2;}
  state CellBalance(index) [function]
    (default) -> (junction 38) : % If_else
    (junction 38) -> (junction 39) [order 1] : [BalanceEn == 1 && (Voltage_mV(i)>(mV_min+Thresholds.Balancing_MaxAllowedImb_mV))]
    (junction 38) -> (junction 40) [order 2] : {BalanceCmd(i)=0;
        | BalanceFetCmd(i,0)}
    (junction 39) -> (junction 41) : {BalanceCmd(i)=1;
        | BalanceFetCmd(i,1)}
    (junction 41) -> (junction 40)
    (junction 40) -> (junction 42)
  Lobby -> Terminate [order 1] : [duration(BalanceEn==0,msec)>Thresholds.Balancing_StateRestPeriod_msec]
  (default) -> Lobby
  Terminate -> Lobby : [duration(BalanceEn==1,msec)>Thresholds.Balancing_StateRestPeriod_msec]
  Odd_Balance -> Lobby [order 1] : [after(BalancingTimeOn_msec,msec)]{BalanceCmd(1:nCells_series) =0;}
  Lobby -> Even_Balance [order 2] : [BalanceEn==1 && after(Thresholds.Balancing_StateRestPeriod_msec,msec)]
  Even_Balance -> Terminate [order 2] : [duration(BalanceEn==0,msec)>Thresholds.Balancing_StateRestPeriod_msec]
  Odd_Balance -> Terminate [order 2] : [duration(BalanceEn==0,msec)>Thresholds.Balancing_StateRestPeriod_msec]
  Even_Balance -> Odd_Balance [order 1] : [after(BalancingTimeOn_msec,msec)]{BalanceCmd(1:nCells_series) =0;}
  data: index function_input; cmd function_input; index function_input; nCells_series input; BalanceCmd output int8 =int8(zeros(1,nCells_series)); mV_min input; Voltage_mV input; BalanceEn input; Thresholds input; i local; CurrentBalancingState output Enum: BalancingState; BalancingTimeOn_msec input

== stateflow chart v00_0A_0E/CellBalancing/InputProcessing/Chart ==
  state BalancingTimeOn_Default
    entry: BalancingTimeOn_msec = double(Balancing_DefaultBalancingTimeOn_msec);
  state BalancingTimeOn_BasedOnTemp_Activate
    entry: x = double(DataPipeline.TemperatureSenseBus(BalancingTempGroup).T_max);
    during: BalancingTimeOn_msec = double(A*x + B);
  (default) -> BalancingTimeOn_Default
  BalancingTimeOn_Default -> BalancingTimeOn_BasedOnTemp_Activate : [duration(DataPipeline.TemperatureSenseBus(BalancingTempGroup).T_max > BalancingCurrentDerateActivationTemp_C , msec) > BalancingCurrentDerateCheckTime_msec]
  data: DataPipeline input; A input; B input; x local double =1; BalancingTempGroup input double; BalancingTimeOn_msec output double =1; Balancing_DefaultBalancingTimeOn_msec input; BalancingCurrentDerateActivationTemp_C input; BalancingCurrentDerateCheckTime_msec input

== stateflow chart v00_0A_0E/HearbeatMonitoring/Chart ==
  state Hardware_NoError
    entry: HardwareError = ProtectionFlags.NoError;
  state Hardware_YesError
    entry: HardwareError = ProtectionFlags.Error;
  (default) -> Hardware_NoError
  Hardware_NoError -> Hardware_YesError : [duration(Status==0,msec)>=Thresholds.HardwareError_Timeout_msec]
  data: Status input; Thresholds input; HardwareError output
